simulink model "husky_sim_yichu_MPC_test"  (R2019b)
settings: Solver=ode4  StartTime=0.0  StopTime=5  FixedStep=Ts  MaxStep=0.001  RelTol=1e-3
InitFcn:
  | init_model;
values from neighbouring files (symbols this model uses):
  desired_input = [0,0,0,0,0,0,0,0,0,0,0,0]    [control_params_init.m]
  m = getfield(leg,'mass')    [dynamic_test.m]    (also in pen_init.m = link2.mass; test.mat = 2.2337)
  q_BL_K0 = initial_angle(12)    [func_params_ext.m]
  q_BR_K0 = initial_angle(9)    [func_params_ext.m]
  q_FL_K0 = initial_angle(6)    [func_params_ext.m]
  q_FR_K0 = initial_angle(3)    [func_params_ext.m]
undefined symbols (not defined in the file or in its folder): body, femur_left, femur_right, hip_left, hip_right, hipf_ctrl, hips_ctrl, knee_ctrl, link_left, link_right, tarsus_left, tarsus_right, tibia_left, tibia_right, X, Y, Z
libraries: sm_lib x247, nesl_utility x86, simulink x36, Contact_Forces_Lib x20
(part 9 of 9)

== system husky_sim_yichu_MPC_test/Husky_simulator/robot_body/Leg_FR/link_fr ==
  Inertia1 : sm_lib/Body Elements/Inertia  InertiaType=Custom  Mass=link_right.mass  MassUnits=kg  CenterOfMass=[0, 0, 0]  CenterOfMassUnits=m  MomentsOfInertia=link_right.MomentsofInertia  MomentsOfInertiaUnits=kg*m^2  ProductsOfInertia=link_right.ProductsofInertia  ProductsOfInertiaUnits=kg*m^2  GraphicType=None  MarkerShape=Inertia  MarkerSize=20  GraphicVisPropType=SimpleVisualProperties  GraphicDiffuseColor=[0.5 0.5 0.5]  GraphicSpecularColor=[0.5 0.5 0.5 1.0]  GraphicAmbientColor=[0.15 0.15 0.15 1.0]  GraphicEmissiveColor=[0.0 0.0 0.0 1.0]  GraphicShininess=75  GraphicOpacity=1.0
  InertiaOriginTransform : sm_lib/Frames and Transforms/Rigid Transform  TranslationMethod=Cartesian  TranslationStandardOffset=0  TranslationLengthUnit=m  TranslationStandardAxis=+Z  TranslationCartesianOffset=[0.15598, 0.00062829, -1.4132e-10]  TranslationROffset=0  TranslationROffsetUnits=m  TranslationZOffset=0  TranslationZOffsetUnits=m  TranslationThetaOffset=0  TranslationThetaOffsetUnits=deg  RotationMethod=RotationSequence  RotationAngleUnits=deg  RotationStandardAxis=+Z  RotationAngle=0.0  RotationArbitraryAxis=[0 0 1]  FollAlignAxisA=+X  BaseAlignAxisA=+Y  FollAlignAxisB=+Y  BaseAlignAxisB=+Z  RotationSequenceAxes=BaseAxes  RotationSequence=XYZ  RotationSequenceAngles=[0, 0, 0]  RotationSequenceAnglesUnits=rad  RotationMatrix=[1 0 0; 0 1 0; 0 0 1]
  ReferenceFrame : sm_lib/Frames and Transforms/Reference Frame
  Visual : sm_lib/Body Elements/File Solid  ExtGeomFileName=husky/meshes/link_fr.STL  UnitType=Custom  ExtGeomFileUnits=m  StepReaderType=HEX  ExportEntireGeometry=off  InertiaType=Custom  Mass=0  MassUnits=kg  CenterOfMass=[0, 0, 0]  CenterOfMassUnits=m  MomentsOfInertia=[0, 0, 0]  MomentsOfInertiaUnits=kg*m^2  ProductsOfInertia=[0, 0, 0]  ProductsOfInertiaUnits=kg*m^2  BasedOnType=DensityFromFile  Density=1000  DensityUnits=kg/m^3  DoExposeReferenceFrame=on  SerializedFrames=<Frames/>  GraphicType=FromGeometry  MarkerShape=Sphere  MarkerSize=10  GraphicVisPropType=SimpleVisualProperties  GraphicDiffuseColor=[1, 0, 0.5]  GraphicSpecularColor=[0.5 0.5 0.5 1.0]  GraphicAmbientColor=[0.15 0.15 0.15 1.0]  GraphicEmissiveColor=[0.0 0.0 0.0 1.0]  GraphicShininess=75  GraphicOpacity=1
  VisualOriginTransform : sm_lib/Frames and Transforms/Rigid Transform  TranslationMethod=Cartesian  TranslationStandardOffset=0  TranslationLengthUnit=m  TranslationStandardAxis=+Z  TranslationCartesianOffset=[0, 0, 0]  TranslationROffset=0  TranslationROffsetUnits=m  TranslationZOffset=0  TranslationZOffsetUnits=m  TranslationThetaOffset=0  TranslationThetaOffsetUnits=deg  RotationMethod=RotationSequence  RotationAngleUnits=deg  RotationStandardAxis=+Z  RotationAngle=0.0  RotationArbitraryAxis=[0 0 1]  FollAlignAxisA=+X  BaseAlignAxisA=+Y  FollAlignAxisB=+Y  BaseAlignAxisB=+Z  RotationSequenceAxes=BaseAxes  RotationSequence=XYZ  RotationSequenceAngles=[0, 0, 0]  RotationSequenceAnglesUnits=rad  RotationMatrix=[1 0 0; 0 1 0; 0 0 1]
  link1_fr_AxisInvTransform : sm_lib/Frames and Transforms/Rigid Transform  TranslationMethod=Cartesian  TranslationStandardOffset=0  TranslationLengthUnit=m  TranslationStandardAxis=+Z  TranslationCartesianOffset=[0, 0, 0]  TranslationROffset=0  TranslationROffsetUnits=m  TranslationZOffset=0  TranslationZOffsetUnits=m  TranslationThetaOffset=0  TranslationThetaOffsetUnits=deg  RotationMethod=ArbitraryAxis  RotationAngleUnits=rad  RotationStandardAxis=+Z  RotationAngle=1.570796326794897  RotationArbitraryAxis=[1, 0, 0]  FollAlignAxisA=+X  BaseAlignAxisA=+Y  FollAlignAxisB=+Y  BaseAlignAxisB=+Z  RotationSequenceAxes=FollowerAxes  RotationSequence=XYX  RotationSequenceAngles=[0 0 0]  RotationSequenceAnglesUnits=deg  RotationMatrix=[1 0 0; 0 1 0; 0 0 1]
  F : PMIOPort  Side=Left
  connections:
  Inertia1/RConn1 -- InertiaOriginTransform/RConn1
  InertiaOriginTransform/LConn1 -- VisualOriginTransform/LConn1 -- link1_fr_AxisInvTransform/LConn1 -- ReferenceFrame/RConn1
  Visual/RConn1 -- VisualOriginTransform/RConn1
  link1_fr_AxisInvTransform/RConn1 -- F/RConn1

== system husky_sim_yichu_MPC_test/Husky_simulator/robot_body/Leg_FR/tarsus_fr ==
  Inertia1 : sm_lib/Body Elements/Inertia  InertiaType=Custom  Mass=tarsus_right.mass  MassUnits=kg  CenterOfMass=[0, 0, 0]  CenterOfMassUnits=m  MomentsOfInertia=tarsus_right.MomentsofInertia  MomentsOfInertiaUnits=kg*m^2  ProductsOfInertia=tarsus_right.ProductsofInertia  ProductsOfInertiaUnits=kg*m^2  GraphicType=None  MarkerShape=Inertia  MarkerSize=20  GraphicVisPropType=SimpleVisualProperties  GraphicDiffuseColor=[0.5 0.5 0.5]  GraphicSpecularColor=[0.5 0.5 0.5 1.0]  GraphicAmbientColor=[0.15 0.15 0.15 1.0]  GraphicEmissiveColor=[0.0 0.0 0.0 1.0]  GraphicShininess=75  GraphicOpacity=1.0
  InertiaOriginTransform : sm_lib/Frames and Transforms/Rigid Transform  TranslationMethod=Cartesian  TranslationStandardOffset=0  TranslationLengthUnit=m  TranslationStandardAxis=+Z  TranslationCartesianOffset=tarsus_right.pCOM  TranslationROffset=0  TranslationROffsetUnits=m  TranslationZOffset=0  TranslationZOffsetUnits=m  TranslationThetaOffset=0  TranslationThetaOffsetUnits=deg  RotationMethod=RotationSequence  RotationAngleUnits=deg  RotationStandardAxis=+Z  RotationAngle=0.0  RotationArbitraryAxis=[0 0 1]  FollAlignAxisA=+X  BaseAlignAxisA=+Y  FollAlignAxisB=+Y  BaseAlignAxisB=+Z  RotationSequenceAxes=BaseAxes  RotationSequence=XYZ  RotationSequenceAngles=[0, 0, 0]  RotationSequenceAnglesUnits=rad  RotationMatrix=[1 0 0; 0 1 0; 0 0 1]
  ReferenceFrame : sm_lib/Frames and Transforms/Reference Frame
  Visual : sm_lib/Body Elements/File Solid  ExtGeomFileName=husky/meshes/tarsus_fr.STL  UnitType=Custom  ExtGeomFileUnits=m  StepReaderType=HEX  ExportEntireGeometry=off  InertiaType=Custom  Mass=0  MassUnits=kg  CenterOfMass=[0, 0, 0]  CenterOfMassUnits=m  MomentsOfInertia=[0, 0, 0]  MomentsOfInertiaUnits=kg*m^2  ProductsOfInertia=[0, 0, 0]  ProductsOfInertiaUnits=kg*m^2  BasedOnType=DensityFromFile  Density=1000  DensityUnits=kg/m^3  DoExposeReferenceFrame=on  SerializedFrames=<Frames/>  GraphicType=FromGeometry  MarkerShape=Sphere  MarkerSize=10  GraphicVisPropType=SimpleVisualProperties  GraphicDiffuseColor=[0.6 1.0 1.0]  GraphicSpecularColor=[0.5 0.5 0.5 1.0]  GraphicAmbientColor=[0.15 0.15 0.15 1.0]  GraphicEmissiveColor=[0.0 0.0 0.0 1.0]  GraphicShininess=75  GraphicOpacity=1
  VisualOriginTransform : sm_lib/Frames and Transforms/Rigid Transform  TranslationMethod=Cartesian  TranslationStandardOffset=0  TranslationLengthUnit=m  TranslationStandardAxis=+Z  TranslationCartesianOffset=[0, 0, 0]  TranslationROffset=0  TranslationROffsetUnits=m  TranslationZOffset=0  TranslationZOffsetUnits=m  TranslationThetaOffset=0  TranslationThetaOffsetUnits=deg  RotationMethod=RotationSequence  RotationAngleUnits=deg  RotationStandardAxis=+Z  RotationAngle=0.0  RotationArbitraryAxis=[0 0 1]  FollAlignAxisA=+X  BaseAlignAxisA=+Y  FollAlignAxisB=+Y  BaseAlignAxisB=+Z  RotationSequenceAxes=BaseAxes  RotationSequence=XYZ  RotationSequenceAngles=[0, 0, 0]  RotationSequenceAnglesUnits=rad  RotationMatrix=[1 0 0; 0 1 0; 0 0 1]
  ankle_fr_AxisInvTransform : sm_lib/Frames and Transforms/Rigid Transform  TranslationMethod=Cartesian  TranslationStandardOffset=0  TranslationLengthUnit=m  TranslationStandardAxis=+Z  TranslationCartesianOffset=[0, 0, 0]  TranslationROffset=0  TranslationROffsetUnits=m  TranslationZOffset=0  TranslationZOffsetUnits=m  TranslationThetaOffset=0  TranslationThetaOffsetUnits=deg  RotationMethod=ArbitraryAxis  RotationAngleUnits=rad  RotationStandardAxis=+Z  RotationAngle=1.570796326794897  RotationArbitraryAxis=[1, 0, 0]  FollAlignAxisA=+X  BaseAlignAxisA=+Y  FollAlignAxisB=+Y  BaseAlignAxisB=+Z  RotationSequenceAxes=FollowerAxes  RotationSequence=XYX  RotationSequenceAngles=[0 0 0]  RotationSequenceAnglesUnits=deg  RotationMatrix=[1 0 0; 0 1 0; 0 0 1]
  foot_contact : sm_lib/Frames and Transforms/Rigid Transform  TranslationMethod=Cartesian  TranslationStandardOffset=0  TranslationLengthUnit=m  TranslationStandardAxis=+Z  TranslationCartesianOffset=[0 0 -0.12]  TranslationROffset=0  TranslationROffsetUnits=m  TranslationZOffset=0  TranslationZOffsetUnits=m  TranslationThetaOffset=0  TranslationThetaOffsetUnits=deg  RotationMethod=RotationSequence  RotationAngleUnits=deg  RotationStandardAxis=+Z  RotationAngle=0.0  RotationArbitraryAxis=[0 0 1]  FollAlignAxisA=+X  BaseAlignAxisA=+Y  FollAlignAxisB=+Y  BaseAlignAxisB=+Z  RotationSequenceAxes=BaseAxes  RotationSequence=XYZ  RotationSequenceAngles=[0, 0, 0]  RotationSequenceAnglesUnits=rad  RotationMatrix=[1 0 0; 0 1 0; 0 0 1]
  link1_fr_AxisTransform : sm_lib/Frames and Transforms/Rigid Transform  TranslationMethod=Cartesian  TranslationStandardOffset=0  TranslationLengthUnit=m  TranslationStandardAxis=+Z  TranslationCartesianOffset=[0, 0, 0]  TranslationROffset=0  TranslationROffsetUnits=m  TranslationZOffset=0  TranslationZOffsetUnits=m  TranslationThetaOffset=0  TranslationThetaOffsetUnits=deg  RotationMethod=ArbitraryAxis  RotationAngleUnits=rad  RotationStandardAxis=+Z  RotationAngle=1.570796326794897  RotationArbitraryAxis=[1, 0, 0]  FollAlignAxisA=+X  BaseAlignAxisA=+Y  FollAlignAxisB=+Y  BaseAlignAxisB=+Z  RotationSequenceAxes=FollowerAxes  RotationSequence=XYX  RotationSequenceAngles=[0 0 0]  RotationSequenceAnglesUnits=deg  RotationMatrix=[1 0 0; 0 1 0; 0 0 1]
  link1_fr_OriginTransform : sm_lib/Frames and Transforms/Rigid Transform  TranslationMethod=Cartesian  TranslationStandardOffset=0  TranslationLengthUnit=m  TranslationStandardAxis=+Z  TranslationCartesianOffset=[0, -0.000499999998312267, 0.0599999999998928]  TranslationROffset=0  TranslationROffsetUnits=m  TranslationZOffset=0  TranslationZOffsetUnits=m  TranslationThetaOffset=0  TranslationThetaOffsetUnits=deg  RotationMethod=RotationSequence  RotationAngleUnits=deg  RotationStandardAxis=+Z  RotationAngle=0.0  RotationArbitraryAxis=[0 0 1]  FollAlignAxisA=+X  BaseAlignAxisA=+Y  FollAlignAxisB=+Y  BaseAlignAxisB=+Z  RotationSequenceAxes=BaseAxes  RotationSequence=XYZ  RotationSequenceAngles=[0, 0, 0]  RotationSequenceAnglesUnits=rad  RotationMatrix=[1 0 0; 0 1 0; 0 0 1]
  F : PMIOPort  Side=Left
  F2 : PMIOPort  Port=2  Side=Right
  link : PMIOPort  Port=3  Side=Right
  connections:
  Inertia1/RConn1 -- InertiaOriginTransform/RConn1
  ankle_fr_AxisInvTransform/LConn1 -- link1_fr_OriginTransform/LConn1 -- foot_contact/LConn1 -- VisualOriginTransform/LConn1 -- InertiaOriginTransform/LConn1 -- ReferenceFrame/RConn1
  Visual/RConn1 -- VisualOriginTransform/RConn1
  ankle_fr_AxisInvTransform/RConn1 -- F/RConn1
  foot_contact/RConn1 -- F2/RConn1
  link1_fr_AxisTransform/LConn1 -- link1_fr_OriginTransform/RConn1
  link1_fr_AxisTransform/RConn1 -- link/RConn1

== system husky_sim_yichu_MPC_test/Husky_simulator/robot_body/Leg_FR/tibia_fr ==
  Inertia : sm_lib/Body Elements/Inertia  InertiaType=Custom  Mass=tibia_right.mass  MassUnits=kg  CenterOfMass=[0, 0, 0]  CenterOfMassUnits=m  MomentsOfInertia=tibia_right.MomentsofInertia  MomentsOfInertiaUnits=kg*m^2  ProductsOfInertia=tibia_right.ProductsofInertia  ProductsOfInertiaUnits=kg*m^2  GraphicType=None  MarkerShape=Inertia  MarkerSize=20  GraphicVisPropType=SimpleVisualProperties  GraphicDiffuseColor=[0.5 0.5 0.5]  GraphicSpecularColor=[0.5 0.5 0.5 1.0]  GraphicAmbientColor=[0.15 0.15 0.15 1.0]  GraphicEmissiveColor=[0.0 0.0 0.0 1.0]  GraphicShininess=75  GraphicOpacity=1.0
  InertiaOriginTransform : sm_lib/Frames and Transforms/Rigid Transform  TranslationMethod=Cartesian  TranslationStandardOffset=0  TranslationLengthUnit=m  TranslationStandardAxis=+Z  TranslationCartesianOffset=tibia_right.pCOM  TranslationROffset=0  TranslationROffsetUnits=m  TranslationZOffset=0  TranslationZOffsetUnits=m  TranslationThetaOffset=0  TranslationThetaOffsetUnits=deg  RotationMethod=RotationSequence  RotationAngleUnits=deg  RotationStandardAxis=+Z  RotationAngle=0.0  RotationArbitraryAxis=[0 0 1]  FollAlignAxisA=+X  BaseAlignAxisA=+Y  FollAlignAxisB=+Y  BaseAlignAxisB=+Z  RotationSequenceAxes=BaseAxes  RotationSequence=XYZ  RotationSequenceAngles=[0, 0, 0]  RotationSequenceAnglesUnits=rad  RotationMatrix=[1 0 0; 0 1 0; 0 0 1]
  ReferenceFrame : sm_lib/Frames and Transforms/Reference Frame
  Visual : sm_lib/Body Elements/File Solid  ExtGeomFileName=husky/meshes/tibia_fr.STL  UnitType=Custom  ExtGeomFileUnits=m  StepReaderType=HEX  ExportEntireGeometry=off  InertiaType=Custom  Mass=0  MassUnits=kg  CenterOfMass=[0, 0, 0]  CenterOfMassUnits=m  MomentsOfInertia=[0, 0, 0]  MomentsOfInertiaUnits=kg*m^2  ProductsOfInertia=[0, 0, 0]  ProductsOfInertiaUnits=kg*m^2  BasedOnType=DensityFromFile  Density=1000  DensityUnits=kg/m^3  DoExposeReferenceFrame=on  SerializedFrames=<Frames/>  GraphicType=FromGeometry  MarkerShape=Sphere  MarkerSize=10  GraphicVisPropType=SimpleVisualProperties  GraphicDiffuseColor=[0, 0, 1]  GraphicSpecularColor=[0.5 0.5 0.5 1.0]  GraphicAmbientColor=[0.15 0.15 0.15 1.0]  GraphicEmissiveColor=[0.0 0.0 0.0 1.0]  GraphicShininess=75  GraphicOpacity=1
  VisualOriginTransform : sm_lib/Frames and Transforms/Rigid Transform  TranslationMethod=Cartesian  TranslationStandardOffset=0  TranslationLengthUnit=m  TranslationStandardAxis=+Z  TranslationCartesianOffset=[0, 0, 0]  TranslationROffset=0  TranslationROffsetUnits=m  TranslationZOffset=0  TranslationZOffsetUnits=m  TranslationThetaOffset=0  TranslationThetaOffsetUnits=deg  RotationMethod=RotationSequence  RotationAngleUnits=deg  RotationStandardAxis=+Z  RotationAngle=0.0  RotationArbitraryAxis=[0 0 1]  FollAlignAxisA=+X  BaseAlignAxisA=+Y  FollAlignAxisB=+Y  BaseAlignAxisB=+Z  RotationSequenceAxes=BaseAxes  RotationSequence=XYZ  RotationSequenceAngles=[0, 0, 0]  RotationSequenceAnglesUnits=rad  RotationMatrix=[1 0 0; 0 1 0; 0 0 1]
  ankle_fr_AxisTransform : sm_lib/Frames and Transforms/Rigid Transform  TranslationMethod=Cartesian  TranslationStandardOffset=0  TranslationLengthUnit=m  TranslationStandardAxis=+Z  TranslationCartesianOffset=[0, 0, 0]  TranslationROffset=0  TranslationROffsetUnits=m  TranslationZOffset=0  TranslationZOffsetUnits=m  TranslationThetaOffset=0  TranslationThetaOffsetUnits=deg  RotationMethod=ArbitraryAxis  RotationAngleUnits=rad  RotationStandardAxis=+Z  RotationAngle=1.570796326794897  RotationArbitraryAxis=[1, 0, 0]  FollAlignAxisA=+X  BaseAlignAxisA=+Y  FollAlignAxisB=+Y  BaseAlignAxisB=+Z  RotationSequenceAxes=FollowerAxes  RotationSequence=XYX  RotationSequenceAngles=[0 0 0]  RotationSequenceAnglesUnits=deg  RotationMatrix=[1 0 0; 0 1 0; 0 0 1]
  ankle_fr_OriginTransform : sm_lib/Frames and Transforms/Rigid Transform  TranslationMethod=Cartesian  TranslationStandardOffset=0  TranslationLengthUnit=m  TranslationStandardAxis=+Z  TranslationCartesianOffset=[-0.333, -0.007, 0]  TranslationROffset=0  TranslationROffsetUnits=m  TranslationZOffset=0  TranslationZOffsetUnits=m  TranslationThetaOffset=0  TranslationThetaOffsetUnits=deg  RotationMethod=RotationSequence  RotationAngleUnits=deg  RotationStandardAxis=+Z  RotationAngle=0.0  RotationArbitraryAxis=[0 0 1]  FollAlignAxisA=+X  BaseAlignAxisA=+Y  FollAlignAxisB=+Y  BaseAlignAxisB=+Z  RotationSequenceAxes=BaseAxes  RotationSequence=XYZ  RotationSequenceAngles=[0, 0, 0]  RotationSequenceAnglesUnits=rad  RotationMatrix=[1 0 0; 0 1 0; 0 0 1]
  knee_fr_AxisInvTransform : sm_lib/Frames and Transforms/Rigid Transform  TranslationMethod=Cartesian  TranslationStandardOffset=0  TranslationLengthUnit=m  TranslationStandardAxis=+Z  TranslationCartesianOffset=[0, 0, 0]  TranslationROffset=0  TranslationROffsetUnits=m  TranslationZOffset=0  TranslationZOffsetUnits=m  TranslationThetaOffset=0  TranslationThetaOffsetUnits=deg  RotationMethod=ArbitraryAxis  RotationAngleUnits=rad  RotationStandardAxis=+Z  RotationAngle=1.570796326794897  RotationArbitraryAxis=[1, 0, 0]  FollAlignAxisA=+X  BaseAlignAxisA=+Y  FollAlignAxisB=+Y  BaseAlignAxisB=+Z  RotationSequenceAxes=FollowerAxes  RotationSequence=XYX  RotationSequenceAngles=[0 0 0]  RotationSequenceAnglesUnits=deg  RotationMatrix=[1 0 0; 0 1 0; 0 0 1]
  F : PMIOPort  Side=Left
  F1 : PMIOPort  Port=2  Side=Right
  connections:
  Inertia/RConn1 -- InertiaOriginTransform/RConn1
  InertiaOriginTransform/LConn1 -- ankle_fr_OriginTransform/LConn1 -- knee_fr_AxisInvTransform/LConn1 -- VisualOriginTransform/LConn1 -- ReferenceFrame/RConn1
  Visual/RConn1 -- VisualOriginTransform/RConn1
  ankle_fr_AxisTransform/RConn1 -- F1/RConn1
  ankle_fr_AxisTransform/LConn1 -- ankle_fr_OriginTransform/RConn1
  knee_fr_AxisInvTransform/RConn1 -- F/RConn1

== matlab function husky_sim_yichu_MPC_test/Husky_simulator/sign_conversion1 ==
  data: q_des input size=12; q_des_sign_converted output size=12
% Changes sign on angles to keep with robot sign convention
%
%   Positive input results in
%   hip frontal - rotate CW (away from body)
%   hip sagittal - rotate CW (rotate leg forward relative to initial position)
%   knee - rotate CW (extension)
%
% Input: q_des  desired input angles
%        angles must be in the following order:
%   q_FR_HF
%   q_FR_HS
%   q_FR_K
%   q_FL_HF
%   q_FL_HS
%   q_FL_K
%   q_BR_HF 
%   q_BR_HS
%   q_BR_K 
%   q_BL_HF 
%   q_BL_HS 
%   q_BL_K 
%
%   Where, FR, FL, BR, BL refers to front right, front left, back right,
%          and back left leg respectively
%       HF, HS, K refers to hip frontal, hip sagittal and knee joints
%       respectively
%
% Output: sign corrected desired angles in the same order as above
%
% By Pravin Dangol, 12-30-19, Boston MA
%
function q_des_sign_converted = func_sign_conversion(q_des)

q_des_sign_converted = q_des;

q_des_sign_converted([1,7]) = -q_des([1,7]);

== matlab function husky_sim_yichu_MPC_test/Husky_simulator/sign_conversion2 ==
  data: q_des input size=12; q_des_sign_converted output size=12
% Changes sign on angles to keep with robot sign convention
%
%   Positive input results in
%   hip frontal - rotate CW (away from body)
%   hip sagittal - rotate CW (rotate leg forward relative to initial position)
%   knee - rotate CW (extension)
%
% Input: q_des  desired input angles
%        angles must be in the following order:
%   q_FR_HF
%   q_FR_HS
%   q_FR_K
%   q_FL_HF
%   q_FL_HS
%   q_FL_K
%   q_BR_HF 
%   q_BR_HS
%   q_BR_K 
%   q_BL_HF 
%   q_BL_HS 
%   q_BL_K 
%
%   Where, FR, FL, BR, BL refers to front right, front left, back right,
%          and back left leg respectively
%       HF, HS, K refers to hip frontal, hip sagittal and knee joints
%       respectively
%
% Output: sign corrected desired angles in the same order as above
%
% By Pravin Dangol, 12-30-19, Boston MA
%
function q_des_sign_converted = func_sign_conversion(q_des)

q_des_sign_converted = q_des;
q_des_sign_converted([1,7]) = -q_des([1,7]);

== matlab function husky_sim_yichu_MPC_test/Husky_simulator/sign_conversion3 ==
  data: q_des input size=12; q_des_sign_converted output size=12
% Changes sign on angles to keep with robot sign convention
%
%   Positive input results in
%   hip frontal - rotate CW (away from body)
%   hip sagittal - rotate CW (rotate leg forward relative to initial position)
%   knee - rotate CW (extension)
%
% Input: q_des  desired input angles
%        angles must be in the following order:
%   q_FR_HF
%   q_FR_HS
%   q_FR_K
%   q_FL_HF
%   q_FL_HS
%   q_FL_K
%   q_BR_HF 
%   q_BR_HS
%   q_BR_K 
%   q_BL_HF 
%   q_BL_HS 
%   q_BL_K 
%
%   Where, FR, FL, BR, BL refers to front right, front left, back right,
%          and back left leg respectively
%       HF, HS, K refers to hip frontal, hip sagittal and knee joints
%       respectively
%
% Output: sign corrected desired angles in the same order as above
%
% By Pravin Dangol, 12-30-19, Boston MA
%
function q_des_sign_converted = func_sign_conversion(q_des)

q_des_sign_converted = q_des;

q_des_sign_converted([1,7]) = -q_des([1,7]);

== matlab function husky_sim_yichu_MPC_test/Husky_simulator/foot end from FK /MATLAB Function ==
  data: sensor_input input; foot_end_position output

%seq=FR FL BR BL
%input should be 12x1, output is 12x1
function foot_end_position = foot_end_position_from_FK(sensor_input)
    foot_end_position=zeros(12,1);
%     for ii=1:12
%         eval(['q',num2str(ii),'=sensor_input(',num2str(ii),');']);
%     end
    q1=-sensor_input(1);
    q2=-sensor_input(2);
    q3=-sensor_input(3);
    q4=-sensor_input(4);
    q5=-sensor_input(5);
    q6=-sensor_input(6);
    q7=-sensor_input(7);
    q8=-sensor_input(8);
    q9=-sensor_input(9);
    q10=-sensor_input(10);
    q11=-sensor_input(11);
    q12=-sensor_input(12);
%      p_BL=[0.19745, 0.045, 0]';
%      p_FR=[0.19745, -0.045, 0]';
%     p_FL=[-0.19745, 0.045, 0]';
% %     p_BR=[-0.19745, -0.045, 0]';

%      p_BL=[-4089/20000;...
%  (53*cos(q10))/1000 + 9/200;...
%         -(53*sin(q10))/1000];
%      p_FR=[3809/20000;...
%  - (53*cos(q1))/1000 - 9/200;...
%            (53*sin(q1))/1000];
%     p_BR=[-4089/20000;...
%  - (53*cos(q7))/1000 - 9/200;...
%            (53*sin(q7))/1000;];
%     p_FL=[3809/20000;...
%  (53*cos(q4))/1000 + 9/200;...
%         -(53*sin(q4))/1000];
    
%     p_FR=[(333*sin(q11)*sin(q12))/1000 - (333*cos(q11)*cos(q12))/1000 - (79*sin(q11))/500 - 4089/20000;...
%  (121*cos(q10))/2000 - (79*cos(q11)*sin(q10))/500 + (333*cos(q11)*sin(q10)*sin(q12))/1000 + (333*cos(q12)*sin(q10)*sin(q11))/1000 + 9/200;...
%          (333*cos(q10)*cos(q11)*sin(q12))/1000 - (79*cos(q10)*cos(q11))/500 - (121*sin(q10))/2000 + (333*cos(q10)*cos(q12)*sin(q11))/1000];
%     p_FL=[(333*sin(q5)*sin(q6))/1000 - (333*cos(q5)*cos(q6))/1000 - (79*sin(q5))/500 + 3809/20000;...
%  (121*cos(q4))/2000 - (79*cos(q5)*sin(q4))/500 + (333*cos(q5)*sin(q4)*sin(q6))/1000 + (333*cos(q6)*sin(q4)*sin(q5))/1000 + 9/200;...
%          (333*cos(q4)*cos(q5)*sin(q6))/1000 - (79*cos(q4)*cos(q5))/500 - (121*sin(q4))/2000 + (333*cos(q4)*cos(q6)*sin(q5))/1000];
%    p_BL=[ - (79*sin(q11))/500 - 4089/20000;...
%  (53*cos(q10))/1000 - (79*cos(q11)*sin(q10))/500 + 9/200;...
%        - (53*sin(q10))/1000 - (79*cos(q10)*cos(q11))/500];
%    p_BR=[ - (79*sin(q8))/500 - 4089/20000;...
%  - (53*cos(q7))/1000 - (79*cos(q8)*sin(q7))/500 - 9/200;...
%            (53*sin(q7))/1000 - (79*cos(q7)*cos(q8))/500];
    
    
    p_FR=[ (333*sin(q2)*sin(q3))/1000 - (333*cos(q2)*cos(q3))/1000 - (79*sin(q2))/500 - (3*cos(q3)*(cos(q2)*sin(q3) + cos(q3)*sin(q2)))/25 + (3*sin(q3)*(cos(q2)*cos(q3) - sin(q2)*sin(q3)))/25 + 3809/20000;...
 (3*cos(q3)*(sin(q1)*sin(q2)*sin(q3) - cos(q2)*cos(q3)*sin(q1)))/25 - (79*cos(q2)*sin(q1))/500 - (121*cos(q1))/2000 - (3*sin(q3)*(cos(q2)*sin(q1)*sin(q3) + cos(q3)*sin(q1)*sin(q2)))/25 + (333*cos(q2)*sin(q1)*sin(q3))/1000 + (333*cos(q3)*sin(q1)*sin(q2))/1000 - 9/200;...
         (121*sin(q1))/2000 - (79*cos(q1)*cos(q2))/500 - (3*cos(q3)*(cos(q1)*cos(q2)*cos(q3) - cos(q1)*sin(q2)*sin(q3)))/25 - (3*sin(q3)*(cos(q1)*cos(q2)*sin(q3) + cos(q1)*cos(q3)*sin(q2)))/25 + (333*cos(q1)*cos(q2)*sin(q3))/1000 + (333*cos(q1)*cos(q3)*sin(q2))/1000];
                                                                               
    p_FL=[  (333*sin(q5)*sin(q6))/1000 - (333*cos(q5)*cos(q6))/1000 - (79*sin(q5))/500 - (3*cos(q6)*(cos(q5)*sin(q6) + cos(q6)*sin(q5)))/25 + (3*sin(q6)*(cos(q5)*cos(q6) - sin(q5)*sin(q6)))/25 + 3809/20000;...
 (121*cos(q4))/2000 - (79*cos(q5)*sin(q4))/500 + (3*cos(q6)*(sin(q4)*sin(q5)*sin(q6) - cos(q5)*cos(q6)*sin(q4)))/25 - (3*sin(q6)*(cos(q5)*sin(q4)*sin(q6) + cos(q6)*sin(q4)*sin(q5)))/25 + (333*cos(q5)*sin(q4)*sin(q6))/1000 + (333*cos(q6)*sin(q4)*sin(q5))/1000 + 9/200;...
         (333*cos(q4)*cos(q5)*sin(q6))/1000 - (79*cos(q4)*cos(q5))/500 - (3*cos(q6)*(cos(q4)*cos(q5)*cos(q6) - cos(q4)*sin(q5)*sin(q6)))/25 - (3*sin(q6)*(cos(q4)*cos(q5)*sin(q6) + cos(q4)*cos(q6)*sin(q5)))/25 - (121*sin(q4))/2000 + (333*cos(q4)*cos(q6)*sin(q5))/1000];
                                                                                   
     p_BR=[(333*sin(q8)*sin(q9))/1000 - (333*cos(q8)*cos(q9))/1000 - (79*sin(q8))/500 - (3*cos(q9)*(cos(q8)*sin(q9) + cos(q9)*sin(q8)))/25 + (3*sin(q9)*(cos(q8)*cos(q9) - sin(q8)*sin(q9)))/25 - 4089/20000;...
 (3*cos(q9)*(sin(q7)*sin(q8)*sin(q9) - cos(q8)*cos(q9)*sin(q7)))/25 - (79*cos(q8)*sin(q7))/500 - (121*cos(q7))/2000 - (3*sin(q9)*(cos(q8)*sin(q7)*sin(q9) + cos(q9)*sin(q7)*sin(q8)))/25 + (333*cos(q8)*sin(q7)*sin(q9))/1000 + (333*cos(q9)*sin(q7)*sin(q8))/1000 - 9/200;...
         (121*sin(q7))/2000 - (79*cos(q7)*cos(q8))/500 - (3*cos(q9)*(cos(q7)*cos(q8)*cos(q9) - cos(q7)*sin(q8)*sin(q9)))/25 - (3*sin(q9)*(cos(q7)*cos(q8)*sin(q9) + cos(q7)*cos(q9)*sin(q8)))/25 + (333*cos(q7)*cos(q8)*sin(q9))/1000 + (333*cos(q7)*cos(q9)*sin(q8))/1000];
                                                                                                                         
    p_BL=[(333*sin(q11)*sin(q12))/1000 - (333*cos(q11)*cos(q12))/1000 - (79*sin(q11))/500 - (3*cos(q12)*(cos(q11)*sin(q12) + cos(q12)*sin(q11)))/25 + (3*sin(q12)*(cos(q11)*cos(q12) - sin(q11)*sin(q12)))/25 - 4089/20000;...
 (121*cos(q10))/2000 - (79*cos(q11)*sin(q10))/500 + (3*cos(q12)*(sin(q10)*sin(q11)*sin(q12) - cos(q11)*cos(q12)*sin(q10)))/25 - (3*sin(q12)*(cos(q11)*sin(q10)*sin(q12) + cos(q12)*sin(q10)*sin(q11)))/25 + (333*cos(q11)*sin(q10)*sin(q12))/1000 + (333*cos(q12)*sin(q10)*sin(q11))/1000 + 9/200;...
         (333*cos(q10)*cos(q11)*sin(q12))/1000 - (79*cos(q10)*cos(q11))/500 - (3*cos(q12)*(cos(q10)*cos(q11)*cos(q12) - cos(q10)*sin(q11)*sin(q12)))/25 - (3*sin(q12)*(cos(q10)*cos(q11)*sin(q12) + cos(q10)*cos(q12)*sin(q11)))/25 - (121*sin(q10))/2000 + (333*cos(q10)*cos(q12)*sin(q11))/1000];
%     p_FR=p_foot_end_FR(sensor_input(1:3));
%     p_FL=p_foot_end_FL(sensor_input(4:6));
%     p_BR=p_foot_end_BR(sensor_input(7:9));
%     p_BL=p_foot_end_BL(sensor_input(10:12));
%     p_FR=subs(p_foot_end_FR,[q1,q2,q3],sensor_input(1:3));
%     p_FL=subs(p_foot_end_FL,[q4,q5,q6],sensor_input(4:6));
%     p_BR=subs(p_foot_end_BR,[q7,q8,q9],sensor_input(7:9));
%     p_BL=subs(p_foot_end_BL,[q10,q11,q12],sensor_input(10:12));
%     foot_end_position=[p_FR(1:3);p_FL(1:3);p_BR(1:3);p_BL(1:3)];
    foot_end_position=[p_FR;p_FL;p_BR;p_BL];
end
